simulink model "BuckyWagon_01"  (Simulink 7.5)
settings: Solver=FixedStepDiscrete  StartTime=0.0  StopTime=10.0  RelTol=1e-3
PreLoadFcn:
  | try, eval([bdroot '_setup']); catch, eval('model_setup', ''); end
InitFcn:
  | try, eval([bdroot '_setup']); catch, eval('model_setup', ''); end
undefined symbols (not defined in the file): ECU565, High, Low, miniviewSetup, motohawk_build_version, motohawk_get_faults, motohawk_setup_toolchains, motohawk_trunc_name, motohawk_vardec_config_group, motohawk_vardec_path, tc, True
libraries: MotoHawk_lib x441, simulink x25, motohawk_engine_lib x19, miniview_lib x10, motohawk_control_primitives_lib x8, motohawk_annotations_lib x2
(part 2 of 8)

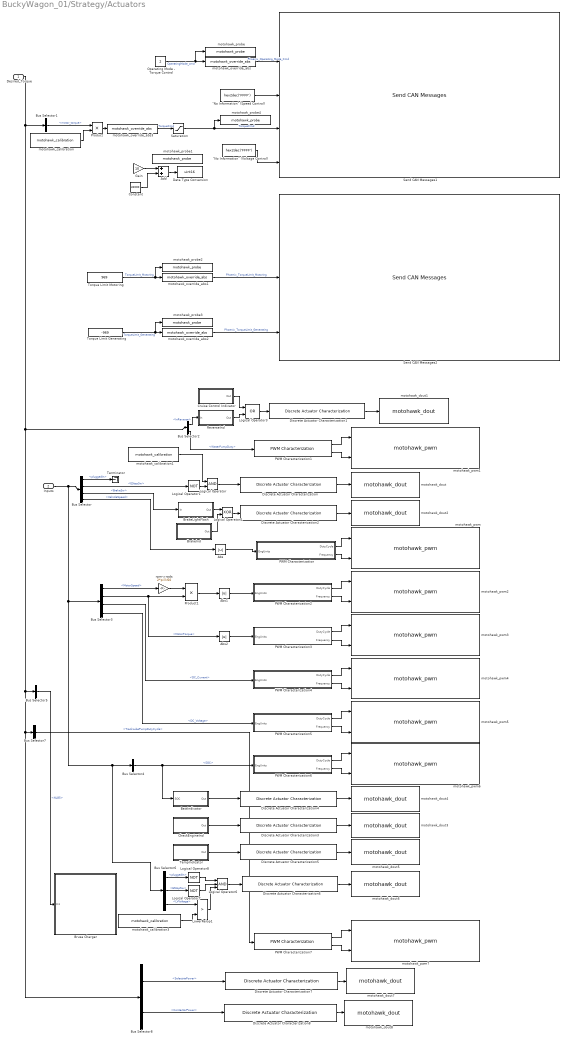
== system BuckyWagon_01/Strategy/Actuators ==
  Desired_Torque : Inport  OutDataType=sfix(16)  OutScaling=2^0
  Inputs : Inport  Port=2  OutDataType=sfix(16)  OutScaling=2^0
  "\"No Information\" (Speed Control)" : Constant  Value=hex2dec('FFFF')  OutDataTypeMode=uint16  OutDataType=sfix(16)  OutScaling=2^0  OutDataTypeStr=uint16
  "\"No Information\" (Voltage Control)" : Constant  Value=hex2dec('FFFF')  OutDataTypeMode=uint16  OutDataType=sfix(16)  OutScaling=2^0  OutDataTypeStr=uint16
  Abs : Abs
  Abs1 : Abs
  Abs2 : Abs
  Add : Sum  OutDataType=fixdt(1, 16)  OutScaling=2^-10
  BattIndicator : Subsystem
  BrakeInd : Subsystem
  BrakeLightFlash : Subsystem
  Brusa Charger : Subsystem  AncestorBlock=motohawk_annotations_lib/Display Image File  mask(Display Image File){image_file='NLG5.jpg'}
      mask prompts: image_file "Image File"
      mask help:
      | Enter an image file on the current MATLAB path to display on this block.
      |
      | Double-clicking this block opens the contents of the subsystem.  Right-click and select 'Mask parameters...' to select a new image file.
      |
      | To use just the mask of this block in a model, but supply your own contents, break the link to the library.
      mask init:
      | try,
      | 	img = imread(image_file);
      | 	motohawk_block_image(gcb, image_file);
      | catch,
      | 	img = imread('image_not_found.jpg');
      | end
      settings: OpenFcn=open_system(gcb,'force');  MoveFcn=motohawk_block_image(gcb, motohawk_get_param_ws(gcb, 'image_file'));
      mask Display: image(img);
  Bus Selector : BusSelector  OutputSignals=Physical.NLG5.pluggedIn,Physical.EStopSw,Physical.BrakeSw,Virtual.VehicleSpeed
  Bus Selector1 : BusSelector  OutputSignals=motor_torque
  Bus Selector2 : BusSelector  OutputSignals=InReverse,WaterPumpDuty
  Bus Selector3 : BusSelector  OutputSignals=Physical.MotorSpeed,Physical.MotorTorque,Physical.DC_Current,Physical.DC_Voltage
  Bus Selector4 : BusSelector  OutputSignals=Virtual.SOC
  Bus Selector5 : BusSelector  OutputSignals=NLG5
  Bus Selector6 : BusSelector  OutputSignals=Physical.NLG5.pluggedIn,Physical.EStopSw,Physical.LVVoltage
  Bus Selector7 : BusSelector  OutputSignals=TrackLubePumpDutyCycle
  Bus Selector8 : BusSelector  OutputSignals=SolectriaPower,ContactorPower
  CheckEngineInd : Subsystem
  Constant : Constant  Value=32000  OutDataType=fixdt(1, 16)  OutScaling=2^0
  Cruise Control Indicator : Subsystem
  Data Type Conversion : DataTypeConversion  OutDataTypeMode=uint16  OutDataType=fixdt(1, 16)  OutScaling=2^0  OutDataTypeStr=uint16
  Discrete Actuator Characterization : motohawk_engine_lib/Discrete Actuator Characterization  SystemSampleTime=-1  prefix='MC_En_'  nam='MC_Enable'  units='bool'  parent_group='Actuators | MC_Enable'  polarity=High-True
  Discrete Actuator Characterization1 : motohawk_engine_lib/Discrete Actuator Characterization  SystemSampleTime=-1  prefix='RevOut_'  nam='ReverseOut'  units='bool'  parent_group='Actuators | Reverse'  polarity=High-True
  Discrete Actuator Characterization2 : motohawk_engine_lib/Discrete Actuator Characterization  SystemSampleTime=-1  prefix='BrkOut_'  nam='Brake_Out'  units='bool'  parent_group='Actuators | Brake'  polarity=High-True
  Discrete Actuator Characterization3 : motohawk_engine_lib/Discrete Actuator Characterization  SystemSampleTime=-1  prefix='ChkEngInd_'  nam='ChkEngInd'  units='bool'  parent_group='Actuators | ChkEngInd'  polarity=High-True
  Discrete Actuator Characterization4 : motohawk_engine_lib/Discrete Actuator Characterization  SystemSampleTime=-1  prefix='BattInd_'  nam='BattInd'  units='bool'  parent_group='Actuators | BattInd'  polarity=High-True
  Discrete Actuator Characterization5 : motohawk_engine_lib/Discrete Actuator Characterization  SystemSampleTime=-1  prefix='TempInd_'  nam='TempInd'  units='bool'  parent_group='Actuators | TempInd'  polarity=High-True
  Discrete Actuator Characterization6 : motohawk_engine_lib/Discrete Actuator Characterization  SystemSampleTime=-1  prefix='ChassisPowerRelayDriver_'  nam='ChassisPowerRelayDriver'  units='bool'  parent_group='Actuators | Chasis Power Relay Driver'  polarity=High-True
  Discrete Actuator Characterization7 : motohawk_engine_lib/Discrete Actuator Characterization  SystemSampleTime=-1  prefix='Solectria_Power_LSD_'  nam='Solectria_Power_LSD'  units='bool'  parent_group='Actuators | Solectria Power LSD'  polarity=Low-True
  Discrete Actuator Characterization8 : motohawk_engine_lib/Discrete Actuator Characterization  SystemSampleTime=-1  prefix='Contactor_Power_LSD_'  nam='Contactor_Power_LSD'  units='bool'  parent_group='Actuators | Contactor Power LSD'  polarity=Low-True
  Gain : Gain  Gain=10  ParameterDataType=fixdt(1, 16)  ParameterScaling=2^0  OutDataType=fixdt(1, 16)  OutScaling=2^0
  Logical Operator : Logic  AllPortsSameDT=off  OutDataTypeMode=boolean  OutDataTypeStr=boolean
  Logical Operator1 : Logic  Operator=NOT  AllPortsSameDT=off  OutDataTypeMode=boolean  OutDataTypeStr=boolean
  Logical Operator3 : Logic  Operator=OR  IconShape=distinctive  AllPortsSameDT=off  OutDataTypeMode=boolean  OutDataTypeStr=boolean
  Logical Operator4 : Logic  Operator=XOR  AllPortsSameDT=off  OutDataTypeMode=boolean  OutDataTypeStr=boolean
  Logical Operator6 : Logic  Inputs=3  AllPortsSameDT=off  OutDataTypeMode=boolean  OutDataTypeStr=boolean
  Logical Operator7 : Logic  Operator=NOT  AllPortsSameDT=off  OutDataTypeMode=boolean  OutDataTypeStr=boolean
  Logical Operator8 : Logic  Operator=NOT  AllPortsSameDT=off  OutDataTypeMode=boolean  OutDataTypeStr=boolean
  LowerRelop1 : RelationalOperator  Operator=>  LogicOutDataTypeMode=boolean  OutDataTypeStr=boolean
  Operating Mode - Torque Control : Constant  Value=2  OutDataType=sfix(16)  OutScaling=2^0
  PWM Characterization : Subsystem  AncestorBlock=motohawk_engine_lib/PWM Characterization  mask(Linear Actuator Characterization){nam='SpeedOut', prefix='SpdOut_', units='mph', parent_group='Actuators | Speed'}
      mask prompts: nam "Name"; parent_group "MotoTune Group"
      mask help:
      | Scales the duty cycle of a PWM signal using a Gain and Offset with a calibratable PWM Frequency.
      | Saturates the converted value around Min and Max values, and converts the signal to the appropriate fixed-point format for use with motoHawk PWM blocks.
      mask init:
      | lbl = ['PWM Characterization: ' nam ];
      | group = [parent_group ' | ' nam];
      settings: RTWSystemCode=Function  RTWFcnNameOpts=Use subsystem name  RTWFileNameOpts=Use function name
      mask Display:
      | patch([0 0 1 1], [0 0.075 0.075 0], [230/255 0/255 0/255])
      | patch([0 0 1 1], [0.025 0.05 0.05 0.025], [150/255 0/255 0/255])
      | patch([0 0 1 1], [0 0.025 0.025 0], [0/255 0/255 0/255])
      | 
      | disp(lbl);
  PWM Characterization1 : motohawk_engine_lib/PWM Characterization  SystemSampleTime=-1  nam='WaterPumpOut'  prefix='WtrPmpOut_'  units='%'  parent_group='Actuators | WaterPump'
  PWM Characterization2 : Subsystem  AncestorBlock=motohawk_engine_lib/PWM Characterization  mask(Linear Actuator Characterization){nam='PowerOut', prefix='PwrOut_', units='W', parent_group='Actuators | Power'}
      mask prompts: nam "Name"; parent_group "MotoTune Group"
      mask help:
      | Scales the duty cycle of a PWM signal using a Gain and Offset with a calibratable PWM Frequency.
      | Saturates the converted value around Min and Max values, and converts the signal to the appropriate fixed-point format for use with motoHawk PWM blocks.
      mask init:
      | lbl = ['PWM Characterization: ' nam ];
      | group = [parent_group ' | ' nam];
      settings: RTWSystemCode=Function  RTWFcnNameOpts=Use subsystem name  RTWFileNameOpts=Use function name
      mask Display:
      | patch([0 0 1 1], [0 0.075 0.075 0], [230/255 0/255 0/255])
      | patch([0 0 1 1], [0.025 0.05 0.05 0.025], [150/255 0/255 0/255])
      | patch([0 0 1 1], [0 0.025 0.025 0], [0/255 0/255 0/255])
      | 
      | disp(lbl);
  PWM Characterization3 : Subsystem  AncestorBlock=motohawk_engine_lib/PWM Characterization  mask(Linear Actuator Characterization){nam='TorqueOut', prefix='TrqOut_', units='Nm', parent_group='Actuators | Torque'}
      mask prompts: nam "Name"; parent_group "MotoTune Group"
      mask help:
      | Scales the duty cycle of a PWM signal using a Gain and Offset with a calibratable PWM Frequency.
      | Saturates the converted value around Min and Max values, and converts the signal to the appropriate fixed-point format for use with motoHawk PWM blocks.
      mask init:
      | lbl = ['PWM Characterization: ' nam ];
      | group = [parent_group ' | ' nam];
      settings: RTWSystemCode=Function  RTWFcnNameOpts=Use subsystem name  RTWFileNameOpts=Use function name
      mask Display:
      | patch([0 0 1 1], [0 0.075 0.075 0], [230/255 0/255 0/255])
      | patch([0 0 1 1], [0.025 0.05 0.05 0.025], [150/255 0/255 0/255])
      | patch([0 0 1 1], [0 0.025 0.025 0], [0/255 0/255 0/255])
      | 
      | disp(lbl);
  PWM Characterization4 : Subsystem  AncestorBlock=motohawk_engine_lib/PWM Characterization  mask(Linear Actuator Characterization){nam='CurrentOut', prefix='CrntOut_', units='A', parent_group='Actuators | Current'}
      mask prompts: nam "Name"; parent_group "MotoTune Group"
      mask help:
      | Scales the duty cycle of a PWM signal using a Gain and Offset with a calibratable PWM Frequency.
      | Saturates the converted value around Min and Max values, and converts the signal to the appropriate fixed-point format for use with motoHawk PWM blocks.
      mask init:
      | lbl = ['PWM Characterization: ' nam ];
      | group = [parent_group ' | ' nam];
      settings: RTWSystemCode=Function  RTWFcnNameOpts=Use subsystem name  RTWFileNameOpts=Use function name
      mask Display:
      | patch([0 0 1 1], [0 0.075 0.075 0], [230/255 0/255 0/255])
      | patch([0 0 1 1], [0.025 0.05 0.05 0.025], [150/255 0/255 0/255])
      | patch([0 0 1 1], [0 0.025 0.025 0], [0/255 0/255 0/255])
      | 
      | disp(lbl);
  PWM Characterization5 : Subsystem  AncestorBlock=motohawk_engine_lib/PWM Characterization  mask(Linear Actuator Characterization){nam='VoltageOut', prefix='VltOut_', units='V', parent_group='Actuators | Voltage'}
      mask prompts: nam "Name"; parent_group "MotoTune Group"
      mask help:
      | Scales the duty cycle of a PWM signal using a Gain and Offset with a calibratable PWM Frequency.
      | Saturates the converted value around Min and Max values, and converts the signal to the appropriate fixed-point format for use with motoHawk PWM blocks.
      mask init:
      | lbl = ['PWM Characterization: ' nam ];
      | group = [parent_group ' | ' nam];
      settings: RTWSystemCode=Function  RTWFcnNameOpts=Use subsystem name  RTWFileNameOpts=Use function name
      mask Display:
      | patch([0 0 1 1], [0 0.075 0.075 0], [230/255 0/255 0/255])
      | patch([0 0 1 1], [0.025 0.05 0.05 0.025], [150/255 0/255 0/255])
      | patch([0 0 1 1], [0 0.025 0.025 0], [0/255 0/255 0/255])
      | 
      | disp(lbl);
  PWM Characterization6 : Subsystem  AncestorBlock=motohawk_engine_lib/PWM Characterization  mask(Linear Actuator Characterization){nam='SOCOut', prefix='SOCOut_', units='%', parent_group='Actuators | SOC'}
      mask prompts: nam "Name"; parent_group "MotoTune Group"
      mask help:
      | Scales the duty cycle of a PWM signal using a Gain and Offset with a calibratable PWM Frequency.
      | Saturates the converted value around Min and Max values, and converts the signal to the appropriate fixed-point format for use with motoHawk PWM blocks.
      mask init:
      | lbl = ['PWM Characterization: ' nam ];
      | group = [parent_group ' | ' nam];
      settings: RTWSystemCode=Function  RTWFcnNameOpts=Use subsystem name  RTWFileNameOpts=Use function name
      mask Display:
      | patch([0 0 1 1], [0 0.075 0.075 0], [230/255 0/255 0/255])
      | patch([0 0 1 1], [0.025 0.05 0.05 0.025], [150/255 0/255 0/255])
      | patch([0 0 1 1], [0 0.025 0.025 0], [0/255 0/255 0/255])
      | 
      | disp(lbl);
  PWM Characterization7 : motohawk_engine_lib/PWM Characterization  SystemSampleTime=-1  nam='TrackLubePumpOut'  prefix='TrackLubePumpOut_'  units='%'  parent_group='Actuators | TrackLubePump'
  Product : Product  OutDataType=sfix(16)  OutScaling=2^0  RndMeth=Zero
  Product1 : Product  OutDataType=sfix(16)  OutScaling=2^0  RndMeth=Zero
  ReverseInd : Subsystem
  Saturation : Saturate  UpperLimit=+3200  LowerLimit=-3200  OutDataType=fixdt(1, 16)  OutScaling=2^0
  Send CAN Messages1 : MotoHawk_lib/CAN Blocks/Send CAN Messages  bus=-2  nam='CAN_1'  msgl=J1939_F9_Control1  pace=5  labelwires=off
  Send CAN Messages2 : MotoHawk_lib/CAN Blocks/Send CAN Messages  bus=-2  nam='CAN_1'  msgl=J1939_F9_Control2  pace=5  labelwires=off
  TempIndicator : Subsystem
  Terminator : Terminator
  Torque Limit Generating : Constant  Value=-969  OutDataType=sfix(16)  OutScaling=2^0
  Torque Limit Motoring : Constant  Value=969  OutDataType=sfix(16)  OutScaling=2^0
  motohawk_calibration : MotoHawk_lib/Calibration & Probing Blocks/motohawk_calibration  nam='MaxTorque'  val=120  storage=Calibration  show_more=on  name_source=Use Parameter  data_type=Inherit from 'Default Value'  read_level=1  write_level=1  ovr_cals=on  view_as=Number  enum_struct={'Disabled', 'Enabled'}  vector_style=Wide Row  use_help_units=off  help=''  units=''  use_header_enum=off  row_header_enum={}  col_header_enum={}  use_min_max=off  min_val=-inf  max_val=inf  use_precision=off  precision=''  gain=1  offset=0  exp=1  use_mototune_group=on  mototune_group='Actuators | Phoenix'
  motohawk_calibration1 : MotoHawk_lib/Calibration & Probing Blocks/motohawk_calibration  nam='MC_Enable'  val=0  storage=Calibration  show_more=on  name_source=Use Parameter  data_type=int8  read_level=1  write_level=1  ovr_cals=on  view_as=Enumeration  enum_struct={'Disabled', 'Enabled'}  vector_style=Wide Row  use_help_units=off  help=''  units=''  use_header_enum=off  row_header_enum={}  col_header_enum={}  use_min_max=off  min_val=-inf  max_val=inf  use_precision=off  precision=''  gain=1  offset=0  exp=1  use_mototune_group=off  mototune_group=motohawk_vardec_path(gcb)
  motohawk_calibration3 : MotoHawk_lib/Calibration & Probing Blocks/motohawk_calibration  nam='ChassisPower_MinSysVolt'  val=12  storage=Calibration  show_more=on  name_source=Use Parameter  data_type=Inherit from 'Default Value'  read_level=1  write_level=1  ovr_cals=on  view_as=Number  enum_struct={'Disabled', 'Enabled'}  vector_style=Wide Row  use_help_units=on  help='Minimum system voltage to turn on chassis power'  units='V'  use_header_enum=off  row_header_enum={}  col_header_enum={}  use_min_max=on  min_val=2  max_val=20  use_precision=on  precision='1.0'  gain=1  offset=0  exp=1  use_mototune_group=on  mototune_group='ESled_11 | Actuators | Chassis Power Relay Driver'
  motohawk_dout : MotoHawk_lib/Digital I//O Blocks/motohawk_dout  resource_name=[]  text_resource=(None)  target=ECU565-128  use_diag=off  use_vardec=on  nam='MC_Enable_Pin'  read_level=1  write_level=1  group='System | I/O Pins | Outputs Config'
  motohawk_dout1 : MotoHawk_lib/Digital I//O Blocks/motohawk_dout  resource_name=[]  text_resource=(None)  target=ECU565-128  use_diag=off  use_vardec=on  nam='ReverseOut_Pin'  read_level=1  write_level=1  group='System | I/O Pins | Outputs Config'
  motohawk_dout2 : MotoHawk_lib/Digital I//O Blocks/motohawk_dout  resource_name=[]  text_resource=(None)  target=ECU565-128  use_diag=off  use_vardec=on  nam='BrakeOut_Pin'  read_level=1  write_level=1  group='System | I/O Pins | Outputs Config'
  motohawk_dout3 : MotoHawk_lib/Digital I//O Blocks/motohawk_dout  resource_name=[]  text_resource=(None)  target=ECU565-128  use_diag=off  use_vardec=on  nam='ChkEngInd_Pin'  read_level=1  write_level=1  group='System | I/O Pins | Outputs Config'
  motohawk_dout4 : MotoHawk_lib/Digital I//O Blocks/motohawk_dout  resource_name=[]  text_resource=(None)  target=ECU565-128  use_diag=off  use_vardec=on  nam='BattInd_Pin'  read_level=1  write_level=1  group='System | I/O Pins | Outputs Config'
  motohawk_dout5 : MotoHawk_lib/Digital I//O Blocks/motohawk_dout  resource_name=[]  text_resource=(None)  target=ECU565-128  use_diag=off  use_vardec=on  nam='TempInd_Pin'  read_level=1  write_level=1  group='System | I/O Pins | Outputs Config'
  motohawk_dout6 : MotoHawk_lib/Digital I//O Blocks/motohawk_dout  resource_name=[]  text_resource=(None)  target=ECU565-128  use_diag=off  use_vardec=on  nam='ChassisPowerRelayDriver_Pin'  read_level=1  write_level=1  group='System | I/O Pins | Outputs Config'
  motohawk_dout7 : MotoHawk_lib/Digital I//O Blocks/motohawk_dout  resource_name=[]  text_resource=(None)  target=ECU565-128  use_diag=off  use_vardec=on  nam='SolectriaPowerLSD_Pin'  read_level=1  write_level=1  group='System | I/O Pins | Outputs Config'
  motohawk_dout8 : MotoHawk_lib/Digital I//O Blocks/motohawk_dout  resource_name=[]  text_resource=(None)  target=ECU565-128  use_diag=off  use_vardec=on  nam='ContactorPowerLSD_Pin'  read_level=1  write_level=1  group='System | I/O Pins | Outputs Config'
  motohawk_override_abs : MotoHawk_lib/Calibration & Probing Blocks/motohawk_override_abs  SystemSampleTime=-1  parent_name='Override_Absolute'  parent_val=0  show_more=on  name_source=Use Output Wire Name  parent_read_level=1  parent_override_level=1  view_as=Number  enum_struct={'Disabled', 'Enabled'}  use_help_units=off  parent_help=''  parent_units=''  use_min_max=off  parent_min=-inf  parent_max=inf  use_precision=off  parent_precision=''  parent_gain=1  parent_offset=0  parent_exp=1  use_mototune_group=on  parent_group='Actuators | Phoenix'
  motohawk_override_abs1 : MotoHawk_lib/Calibration & Probing Blocks/motohawk_override_abs  SystemSampleTime=-1  parent_name='Override_Absolute'  parent_val=0  show_more=on  name_source=Use Output Wire Name  parent_read_level=1  parent_override_level=1  view_as=Number  enum_struct={'Disabled', 'Enabled'}  use_help_units=off  parent_help=''  parent_units=''  use_min_max=off  parent_min=-inf  parent_max=inf  use_precision=off  parent_precision=''  parent_gain=1  parent_offset=0  parent_exp=1  use_mototune_group=on  parent_group='Actuators | Phoenix'
  motohawk_override_abs2 : MotoHawk_lib/Calibration & Probing Blocks/motohawk_override_abs  SystemSampleTime=-1  parent_name='Override_Absolute'  parent_val=0  show_more=on  name_source=Use Output Wire Name  parent_read_level=1  parent_override_level=1  view_as=Number  enum_struct={'Disabled', 'Enabled'}  use_help_units=off  parent_help=''  parent_units=''  use_min_max=off  parent_min=-inf  parent_max=inf  use_precision=off  parent_precision=''  parent_gain=1  parent_offset=0  parent_exp=1  use_mototune_group=on  parent_group='Actuators | Phoenix'
  motohawk_override_abs3 : MotoHawk_lib/Calibration & Probing Blocks/motohawk_override_abs  SystemSampleTime=-1  parent_name='TorqueControl'  parent_val=0  show_more=on  name_source=Use Parameter  parent_read_level=1  parent_override_level=1  view_as=Number  enum_struct={'Disabled', 'Enabled'}  use_help_units=off  parent_help=''  parent_units=''  use_min_max=off  parent_min=-inf  parent_max=inf  use_precision=off  parent_precision=''  parent_gain=1  parent_offset=0  parent_exp=1  use_mototune_group=on  parent_group='Actuators | Phoenix'
  motohawk_probe : MotoHawk_lib/Calibration & Probing Blocks/motohawk_probe  nam='Phoenix_Operating_Mode_Command'  show_more=on  name_source=Use Parameter  read_level=1  view_as=Number  enum_struct={'Disabled', 'Enabled'}  vector_style=Wide Row  use_help_units=off  help=''  units=''  use_header_enum=off  row_header_enum={}  col_header_enum={}  use_precision=off  precision=''  gain=1  offset=0  exp=1  use_mototune_group=on  mototune_group='Actuators | Phoenix'
  motohawk_probe1 : MotoHawk_lib/Calibration & Probing Blocks/motohawk_probe  nam='Phoenix_TorqueCmd_integer'  show_more=on  name_source=Use Parameter  read_level=1  view_as=Number  enum_struct={'Disabled', 'Enabled'}  vector_style=Wide Row  use_help_units=off  help=''  units=''  use_header_enum=off  row_header_enum={}  col_header_enum={}  use_precision=off  precision=''  gain=1  offset=0  exp=1  use_mototune_group=on  mototune_group='Actuators | Phoenix'
  motohawk_probe2 : MotoHawk_lib/Calibration & Probing Blocks/motohawk_probe  nam='Phoenix_TorqueLimit_Motoring'  show_more=on  name_source=Use Parameter  read_level=1  view_as=Number  enum_struct={'Disabled', 'Enabled'}  vector_style=Wide Row  use_help_units=off  help=''  units=''  use_header_enum=off  row_header_enum={}  col_header_enum={}  use_precision=off  precision=''  gain=1  offset=0  exp=1  use_mototune_group=on  mototune_group='Actuators | Phoenix'
  motohawk_probe3 : MotoHawk_lib/Calibration & Probing Blocks/motohawk_probe  nam='Phoenix_TorqueLimit_Generating'  show_more=on  name_source=Use Parameter  read_level=1  view_as=Number  enum_struct={'Disabled', 'Enabled'}  vector_style=Wide Row  use_help_units=off  help=''  units=''  use_header_enum=off  row_header_enum={}  col_header_enum={}  use_precision=off  precision=''  gain=1  offset=0  exp=1  use_mototune_group=on  mototune_group='Actuators | Phoenix'
  motohawk_probe4 : MotoHawk_lib/Calibration & Probing Blocks/motohawk_probe  nam='Phoenix_TorqueCmd_final'  show_more=on  name_source=Use Parameter  read_level=1  view_as=Number  enum_struct={'Disabled', 'Enabled'}  vector_style=Wide Row  use_help_units=off  help=''  units=''  use_header_enum=off  row_header_enum={}  col_header_enum={}  use_precision=off  precision=''  gain=1  offset=0  exp=1  use_mototune_group=on  mototune_group='Actuators | Phoenix'
  motohawk_pwm : MotoHawk_lib/Analog I//O Blocks/motohawk_pwm  res_name=[]  text_resource=(None)  code_resource=NONE  val_resource=-1  target=ECU565-128  resource_enum_str=(None)=-1,H1=1,H2=10,FINJ1=12,FINJ2=13,FINJ3=14,FINJ4=15,FINJ5=16,FINJ6=17,FINJ7=18,FINJ8=19,FINJ9=20,FINJ10=21,FINJ11=22,FINJ12=23,TACH=24,LSD1=25,LSD2=26,LSD3=27,LSD4=28,LSD5=29,LSD6=30,LSD7=31,LSD8=32,LSD9=33,LSD10=34,EST 1=36,EST 2=37,EST 3=38,EST 4=39,EST 5=40,EST 6=41,EST 7=42,EST 8=43,EST 9=44,EST 10=45,EST 11=46,EST 12=47,EST 13=48,EST 14=49,EST 15=50,EST 16=51,H3=107  freq_mode=-1  min_freq=2  use_max_freq=off  max_freq=42949672.96  use_enable=off  use_brake=off  output_current=off  output_fault_status=off  use_child=off  use_vardec=on  nam='SpeedOut_Pin'  read_level=1  write_level=1  group='System | I/O Pins | Outputs Config'
  motohawk_pwm1 : MotoHawk_lib/Analog I//O Blocks/motohawk_pwm  res_name=[]  text_resource=(None)  code_resource=NONE  val_resource=-1  target=ECU565-128  resource_enum_str=(None)=-1,H1=1,H2=10,FINJ1=12,FINJ2=13,FINJ3=14,FINJ4=15,FINJ5=16,FINJ6=17,FINJ7=18,FINJ8=19,FINJ9=20,FINJ10=21,FINJ11=22,FINJ12=23,TACH=24,LSD1=25,LSD2=26,LSD3=27,LSD4=28,LSD5=29,LSD6=30,LSD7=31,LSD8=32,LSD9=33,LSD10=34,EST 1=36,EST 2=37,EST 3=38,EST 4=39,EST 5=40,EST 6=41,EST 7=42,EST 8=43,EST 9=44,EST 10=45,EST 11=46,EST 12=47,EST 13=48,EST 14=49,EST 15=50,EST 16=51,H3=107  freq_mode=-1  min_freq=2  use_max_freq=off  max_freq=42949672.96  use_enable=off  use_brake=off  output_current=off  output_fault_status=off  use_child=off  use_vardec=on  nam='WaterPump_Pin'  read_level=1  write_level=1  group='System | I/O Pins | Outputs Config'
  motohawk_pwm2 : MotoHawk_lib/Analog I//O Blocks/motohawk_pwm  res_name=[]  text_resource=(None)  code_resource=NONE  val_resource=-1  target=ECU565-128  resource_enum_str=(None)=-1,H1=1,H2=10,FINJ1=12,FINJ2=13,FINJ3=14,FINJ4=15,FINJ5=16,FINJ6=17,FINJ7=18,FINJ8=19,FINJ9=20,FINJ10=21,FINJ11=22,FINJ12=23,TACH=24,LSD1=25,LSD2=26,LSD3=27,LSD4=28,LSD5=29,LSD6=30,LSD7=31,LSD8=32,LSD9=33,LSD10=34,EST 1=36,EST 2=37,EST 3=38,EST 4=39,EST 5=40,EST 6=41,EST 7=42,EST 8=43,EST 9=44,EST 10=45,EST 11=46,EST 12=47,EST 13=48,EST 14=49,EST 15=50,EST 16=51,H3=107  freq_mode=-1  min_freq=2  use_max_freq=off  max_freq=42949672.96  use_enable=off  use_brake=off  output_current=off  output_fault_status=off  use_child=off  use_vardec=on  nam='PowerOut_Pin'  read_level=1  write_level=1  group='System | I/O Pins | Outputs Config'
  motohawk_pwm3 : MotoHawk_lib/Analog I//O Blocks/motohawk_pwm  res_name=[]  text_resource=(None)  code_resource=NONE  val_resource=-1  target=ECU565-128  resource_enum_str=(None)=-1,H1=1,H2=10,FINJ1=12,FINJ2=13,FINJ3=14,FINJ4=15,FINJ5=16,FINJ6=17,FINJ7=18,FINJ8=19,FINJ9=20,FINJ10=21,FINJ11=22,FINJ12=23,TACH=24,LSD1=25,LSD2=26,LSD3=27,LSD4=28,LSD5=29,LSD6=30,LSD7=31,LSD8=32,LSD9=33,LSD10=34,EST 1=36,EST 2=37,EST 3=38,EST 4=39,EST 5=40,EST 6=41,EST 7=42,EST 8=43,EST 9=44,EST 10=45,EST 11=46,EST 12=47,EST 13=48,EST 14=49,EST 15=50,EST 16=51,H3=107  freq_mode=-1  min_freq=2  use_max_freq=off  max_freq=42949672.96  use_enable=off  use_brake=off  output_current=off  output_fault_status=off  use_child=off  use_vardec=on  nam='TorqueOut_Pin'  read_level=1  write_level=1  group='System | I/O Pins | Outputs Config'
  motohawk_pwm4 : MotoHawk_lib/Analog I//O Blocks/motohawk_pwm  res_name=[]  text_resource=(None)  code_resource=NONE  val_resource=-1  target=ECU565-128  resource_enum_str=(None)=-1,H1=1,H2=10,FINJ1=12,FINJ2=13,FINJ3=14,FINJ4=15,FINJ5=16,FINJ6=17,FINJ7=18,FINJ8=19,FINJ9=20,FINJ10=21,FINJ11=22,FINJ12=23,TACH=24,LSD1=25,LSD2=26,LSD3=27,LSD4=28,LSD5=29,LSD6=30,LSD7=31,LSD8=32,LSD9=33,LSD10=34,EST 1=36,EST 2=37,EST 3=38,EST 4=39,EST 5=40,EST 6=41,EST 7=42,EST 8=43,EST 9=44,EST 10=45,EST 11=46,EST 12=47,EST 13=48,EST 14=49,EST 15=50,EST 16=51,H3=107  freq_mode=-1  min_freq=2  use_max_freq=off  max_freq=42949672.96  use_enable=off  use_brake=off  output_current=off  output_fault_status=off  use_child=off  use_vardec=on  nam='CurrentOut_Pin'  read_level=1  write_level=1  group='System | I/O Pins | Outputs Config'
  motohawk_pwm5 : MotoHawk_lib/Analog I//O Blocks/motohawk_pwm  res_name=[]  text_resource=(None)  code_resource=NONE  val_resource=-1  target=ECU565-128  resource_enum_str=(None)=-1,H1=1,H2=10,FINJ1=12,FINJ2=13,FINJ3=14,FINJ4=15,FINJ5=16,FINJ6=17,FINJ7=18,FINJ8=19,FINJ9=20,FINJ10=21,FINJ11=22,FINJ12=23,TACH=24,LSD1=25,LSD2=26,LSD3=27,LSD4=28,LSD5=29,LSD6=30,LSD7=31,LSD8=32,LSD9=33,LSD10=34,EST 1=36,EST 2=37,EST 3=38,EST 4=39,EST 5=40,EST 6=41,EST 7=42,EST 8=43,EST 9=44,EST 10=45,EST 11=46,EST 12=47,EST 13=48,EST 14=49,EST 15=50,EST 16=51,H3=107  freq_mode=-1  min_freq=2  use_max_freq=off  max_freq=42949672.96  use_enable=off  use_brake=off  output_current=off  output_fault_status=off  use_child=off  use_vardec=on  nam='VoltageOut_Pin'  read_level=1  write_level=1  group='System | I/O Pins | Outputs Config'
  motohawk_pwm6 : MotoHawk_lib/Analog I//O Blocks/motohawk_pwm  res_name=[]  text_resource=(None)  code_resource=NONE  val_resource=-1  target=ECU565-128  resource_enum_str=(None)=-1,H1=1,H2=10,FINJ1=12,FINJ2=13,FINJ3=14,FINJ4=15,FINJ5=16,FINJ6=17,FINJ7=18,FINJ8=19,FINJ9=20,FINJ10=21,FINJ11=22,FINJ12=23,TACH=24,LSD1=25,LSD2=26,LSD3=27,LSD4=28,LSD5=29,LSD6=30,LSD7=31,LSD8=32,LSD9=33,LSD10=34,EST 1=36,EST 2=37,EST 3=38,EST 4=39,EST 5=40,EST 6=41,EST 7=42,EST 8=43,EST 9=44,EST 10=45,EST 11=46,EST 12=47,EST 13=48,EST 14=49,EST 15=50,EST 16=51,H3=107  freq_mode=-1  min_freq=2  use_max_freq=off  max_freq=42949672.96  use_enable=off  use_brake=off  output_current=off  output_fault_status=off  use_child=off  use_vardec=on  nam='SOCOut_Pin'  read_level=1  write_level=1  group='System | I/O Pins | Outputs Config'
  motohawk_pwm7 : MotoHawk_lib/Analog I//O Blocks/motohawk_pwm  res_name=[]  text_resource=(None)  code_resource=NONE  val_resource=-1  target=ECU565-128  resource_enum_str=(None)=-1,H1=1,H2=10,FINJ1=12,FINJ2=13,FINJ3=14,FINJ4=15,FINJ5=16,FINJ6=17,FINJ7=18,FINJ8=19,FINJ9=20,FINJ10=21,FINJ11=22,FINJ12=23,TACH=24,LSD1=25,LSD2=26,LSD3=27,LSD4=28,LSD5=29,LSD6=30,LSD7=31,LSD8=32,LSD9=33,LSD10=34,EST 1=36,EST 2=37,EST 3=38,EST 4=39,EST 5=40,EST 6=41,EST 7=42,EST 8=43,EST 9=44,EST 10=45,EST 11=46,EST 12=47,EST 13=48,EST 14=49,EST 15=50,EST 16=51,H3=107  freq_mode=-1  min_freq=2  use_max_freq=off  max_freq=42949672.96  use_enable=off  use_brake=off  output_current=off  output_fault_status=off  use_child=off  use_vardec=on  nam='TrackLubePump_Pin'  read_level=1  write_level=1  group='System | I/O Pins | Outputs Config'
  rpm->rads : Gain  Gain=2*pi()/60  ParameterDataType=sfix(16)  ParameterScaling=2^0  OutDataType=sfix(16)  OutScaling=2^0
  wires:
  motohawk_override_abs/1 -> Send CAN Messages1/2  "Phoenix_Operating_Mode_Cmd"
  Operating Mode - Torque Control/1 -> motohawk_override_abs/1, motohawk_probe/1  "OperatingMode_cmd"
  motohawk_calibration/1 -> Product/2
  Product/1 -> motohawk_override_abs3/1
  Discrete Actuator Characterization/1 -> motohawk_dout/1
  Inputs/1 -> Bus Selector/1, Bus Selector3/1, Bus Selector4/1, Bus Selector6/1
  Logical Operator/1 -> Discrete Actuator Characterization/1
  motohawk_calibration1/1 -> Logical Operator/1
  Bus Selector/2 -> Logical Operator1/1  "<EStopSw>"
  Discrete Actuator Characterization1/1 -> motohawk_dout1/1
  Discrete Actuator Characterization2/1 -> motohawk_dout2/1
  PWM Characterization/1(DutyCycle) -> motohawk_pwm/1
  PWM Characterization/2(Frequency) -> motohawk_pwm/2
  Bus Selector/3 -> BrakeLightFlash/1(In)  "<BrakeSw>"
  Desired_Torque/1 -> Bus Selector1/1, Bus Selector2/1, Bus Selector5/1, Bus Selector7/1, Bus Selector8/1
  Bus Selector1/1 -> Product/1  "<motor_torque>"
  Bus Selector/4 -> Abs/1  "<VehicleSpeed>"
  PWM Characterization1/1 -> motohawk_pwm1/1
  PWM Characterization1/2 -> motohawk_pwm1/2
  Bus Selector2/2 -> PWM Characterization1/1  "<WaterPumpDuty>"
  Logical Operator1/1 -> Logical Operator/2
  PWM Characterization2/1(DutyCycle) -> motohawk_pwm2/1
  PWM Characterization2/2(Frequency) -> motohawk_pwm2/2
  PWM Characterization3/1(DutyCycle) -> motohawk_pwm3/1
  PWM Characterization3/2(Frequency) -> motohawk_pwm3/2
  Bus Selector3/1 -> rpm->rads/1  "<MotorSpeed>"
  rpm->rads/1 -> Product1/1
  Bus Selector3/2 -> Product1/2, Abs2/1  "<MotorTorque>"
  Product1/1 -> Abs1/1
  Discrete Actuator Characterization3/1 -> motohawk_dout3/1
  CheckEngineInd/1(Out) -> Discrete Actuator Characterization3/1
  Discrete Actuator Characterization4/1 -> motohawk_dout4/1
  PWM Characterization4/1(DutyCycle) -> motohawk_pwm4/1
  PWM Characterization4/2(Frequency) -> motohawk_pwm4/2
  PWM Characterization5/1(DutyCycle) -> motohawk_pwm5/1
  PWM Characterization5/2(Frequency) -> motohawk_pwm5/2
  Discrete Actuator Characterization5/1 -> motohawk_dout5/1
  TempIndicator/1(Out) -> Discrete Actuator Characterization5/1
  Bus Selector3/3 -> PWM Characterization4/1(EngUnits)  "<DC_Current>"
  Bus Selector3/4 -> PWM Characterization5/1(EngUnits)  "<DC_Voltage>"
  BattIndicator/1(Out) -> Discrete Actuator Characterization4/1
  Bus Selector4/1 -> BattIndicator/1(SOC), PWM Characterization6/1(EngUnits)  "<SOC>"
  PWM Characterization6/1(DutyCycle) -> motohawk_pwm6/1
  PWM Characterization6/2(Frequency) -> motohawk_pwm6/2
  Abs/1 -> PWM Characterization/1(EngUnits)
  Abs1/1 -> PWM Characterization2/1(EngUnits)
  Abs2/1 -> PWM Characterization3/1(EngUnits)
  Bus Selector2/1 -> ReverseInd/1(In)  "<InReverse>"
  Cruise Control Indicator/1(Out) -> Logical Operator3/1
  ReverseInd/1(Out) -> Logical Operator3/2
  Logical Operator3/1 -> Discrete Actuator Characterization1/1
  Bus Selector5/1 -> Brusa Charger/1(In1)  "<NLG5>"
  BrakeLightFlash/1(Out) -> Logical Operator4/1
  BrakeInd/1(Out) -> Logical Operator4/2
  Logical Operator4/1 -> Discrete Actuator Characterization2/1
  Bus Selector6/1 -> Logical Operator8/1  "<pluggedIn>"
  Bus Selector6/2 -> Logical Operator7/1  "<EStopSw>"
  Logical Operator6/1 -> Discrete Actuator Characterization6/1
  Logical Operator8/1 -> Logical Operator6/1
  Logical Operator7/1 -> Logical Operator6/2
  motohawk_calibration3/1 -> LowerRelop1/2
  Bus Selector6/3 -> LowerRelop1/1  "<LVVoltage>"
  LowerRelop1/1 -> Logical Operator6/3
  Discrete Actuator Characterization6/1 -> motohawk_dout6/1
  PWM Characterization7/1 -> motohawk_pwm7/1
  PWM Characterization7/2 -> motohawk_pwm7/2
  Bus Selector7/1 -> PWM Characterization7/1  "<TrackLubePumpDutyCycle>"
  Discrete Actuator Characterization8/1 -> motohawk_dout8/1
  Discrete Actuator Characterization7/1 -> motohawk_dout7/1
  Bus Selector8/1 -> Discrete Actuator Characterization7/1  "<SolectriaPower>"
  Bus Selector8/2 -> Discrete Actuator Characterization8/1  "<ContactorPower>"
  Bus Selector/1 -> Terminator/1  "<pluggedIn>"
  "\"No Information\" (Speed Control)"/1 -> Send CAN Messages1/3
  "\"No Information\" (Voltage Control)"/1 -> Send CAN Messages1/5
  motohawk_override_abs3/1 -> Saturation/1  "TorqueCmd"
  Saturation/1 -> Send CAN Messages1/4, motohawk_probe4/1  "TorqueCmd"
  motohawk_override_abs1/1 -> Send CAN Messages2/2  "Phoenix_TorqueLimit_Motoring"
  Torque Limit Motoring/1 -> motohawk_probe2/1, motohawk_override_abs1/1  "TorqueLimit_Motoring"
  motohawk_override_abs2/1 -> Send CAN Messages2/3  "Phoenix_TorqueLimit_Generating"
  Torque Limit Generating/1 -> motohawk_override_abs2/1, motohawk_probe3/1  "TorqueLimit_Generating"
  Gain/1 -> Add/1
  Constant/1 -> Add/2
  Add/1 -> Data Type Conversion/1

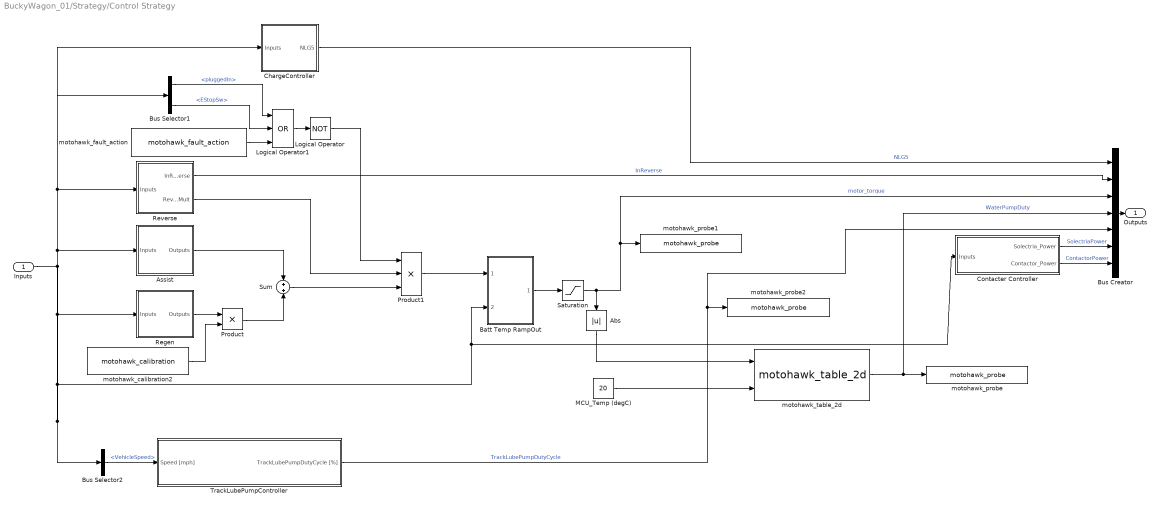
== system BuckyWagon_01/Strategy/Control Strategy ==
  Inputs : Inport  OutDataType=sfix(16)  OutScaling=2^0
  Abs : Abs
  Assist : Subsystem  TreatAsAtomicUnit=on
  Batt Temp RampOut : Subsystem
  Bus Creator : BusCreator  Inputs=7
  Bus Selector1 : BusSelector  OutputSignals=Physical.NLG5.pluggedIn,Physical.EStopSw
  Bus Selector2 : BusSelector  OutputSignals=Virtual.VehicleSpeed
  ChargeController : Subsystem  TreatAsAtomicUnit=on
  Contacter Controller : Subsystem
  Logical Operator : Logic  Operator=NOT  AllPortsSameDT=off  OutDataTypeMode=boolean  OutDataTypeStr=boolean
  Logical Operator1 : Logic  Operator=OR  Inputs=3  AllPortsSameDT=off  OutDataTypeMode=boolean  OutDataTypeStr=boolean
  MCU_Temp (degC) : Constant  Value=20  OutDataType=fixdt(1, 16)  OutScaling=2^0
  Product : Product  OutDataType=sfix(16)  OutScaling=2^0  RndMeth=Zero
  Product1 : Product  Inputs=3  OutDataType=sfix(16)  OutScaling=2^0  RndMeth=Zero
  Regen : Subsystem  TreatAsAtomicUnit=on
  Reverse : Subsystem  TreatAsAtomicUnit=on
  Saturation : Saturate  UpperLimit=1  LowerLimit=-1
  Sum : Sum  OutDataType=sfix(16)  OutScaling=2^0
  TrackLubePumpController : Subsystem  TreatAsAtomicUnit=on
  motohawk_calibration2 : MotoHawk_lib/Calibration & Probing Blocks/motohawk_calibration  nam='Regen_Enable'  val=0  storage=Calibration  show_more=on  name_source=Use Parameter  data_type=Inherit from 'Default Value'  read_level=1  write_level=1  ovr_cals=on  view_as=Number  enum_struct={'Disabled', 'Enabled'}  vector_style=Wide Row  use_help_units=on  help='Enables Regen Braking'  units=''  use_header_enum=off  row_header_enum={}  col_header_enum={}  use_min_max=off  min_val=0  max_val=1  use_precision=on  precision='1.0'  gain=1  offset=0  exp=1  use_mototune_group=off  mototune_group=motohawk_vardec_path(gcb)
  motohawk_fault_action : MotoHawk_lib/Fault Management Blocks/motohawk_fault_action  nam='DisableDrive'  output_status=on  eval_nam=DisableDrive
  motohawk_probe : MotoHawk_lib/Calibration & Probing Blocks/motohawk_probe  nam='WaterPumpDuty'  show_more=off  name_source=Use Parameter  read_level=1  view_as=Number  enum_struct={'Disabled', 'Enabled'}  vector_style=Wide Row  use_help_units=off  help=''  units=''  use_header_enum=off  row_header_enum={}  col_header_enum={}  use_precision=off  precision=''  gain=1  offset=0  exp=1  use_mototune_group=off  mototune_group=motohawk_vardec_path(gcb)
  motohawk_probe1 : MotoHawk_lib/Calibration & Probing Blocks/motohawk_probe  nam='motor_Torque'  show_more=on  name_source=Use Parameter  read_level=1  view_as=Number  enum_struct={'Disabled', 'Enabled'}  vector_style=Wide Row  use_help_units=off  help=''  units=''  use_header_enum=off  row_header_enum={}  col_header_enum={}  use_precision=on  precision='1.3'  gain=1  offset=0  exp=1  use_mototune_group=off  mototune_group=motohawk_vardec_path(gcb)
  motohawk_probe2 : MotoHawk_lib/Calibration & Probing Blocks/motohawk_probe  nam='TrackLubePumpDutyCycle'  show_more=on  name_source=Use Parameter  read_level=1  view_as=Number  enum_struct={'Disabled', 'Enabled'}  vector_style=Wide Row  use_help_units=off  help=''  units=''  use_header_enum=off  row_header_enum={}  col_header_enum={}  use_precision=on  precision='1.3'  gain=1  offset=0  exp=1  use_mototune_group=off  mototune_group=motohawk_vardec_path(gcb)
  motohawk_table_2d : MotoHawk_lib/Lookup Tables/motohawk_table_2d  SystemSampleTime=-1  nam='WaterPumpDutyMap'  row_nam='MotorTorque'  col_nam='MCUTemp'  row_breakpoint_data=0:0.1:1  col_breakpoint_data=0:10:100  table_data=ones(11,11)  show_more=off  row_bp_data_type=Inherit from 'Row Breakpoint Data'  col_bp_data_type=Inherit from 'Column Breakpoint Data'  bp_storage=Constant  table_data_type=Inherit from 'Table Data'  storage=NonAdaptive  read_level=1  write_level=1  ovr_cals=on  use_help=off  help=''  row_bp_units=''  col_bp_units=''  table_units=''  use_min_max=off  row_bp_min_val=-inf  row_bp_max_val=inf  col_bp_min_val=-inf  col_bp_max_val=inf  min_val=-inf  max_val=inf  use_precision=off  use_row_breakpoint=off  rb_precision=''  rb_gain=1  rb_offset=0  rb_exp=1  use_col_breakpoint=off  cb_precision=''  cb_gain=1  cb_offset=0  cb_exp=1  use_table=off  t_precision=''  t_gain=1  t_offset=0  t_exp=1  use_links=off  row_input_name=''  col_input_name=''  output_name=''  use_mototune_group=off  mototune_group=motohawk_vardec_path(gcb)
  Outputs : Outport  OutDataType=sfix(16)  OutScaling=2^0
  wires:
  Inputs/1 -> Assist/1(Inputs), Reverse/1(Inputs), Bus Selector1/1, Regen/1(Inputs), ChargeController/1(Inputs), Bus Selector2/1, Batt Temp RampOut/2(Sensors), Contacter Controller/1(Inputs)
  Saturation/1 -> motohawk_probe1/1, Bus Creator/3, Abs/1  "motor_torque"
  Regen/1(Outputs) -> Product/1
  motohawk_calibration2/1 -> Product/2
  Assist/1(Outputs) -> Sum/1
  Batt Temp RampOut/1(Torque_Out) -> Saturation/1
  Product/1 -> Sum/2
  Reverse/2(ReverseMult) -> Product1/2
  Product1/1 -> Batt Temp RampOut/1(Torque_In)
  Sum/1 -> Product1/3
  Logical Operator/1 -> Product1/1
  Reverse/1(InReverse) -> Bus Creator/2  "InReverse"
  Bus Creator/1 -> Outputs/1
  Abs/1 -> motohawk_table_2d/1
  MCU_Temp (degC)/1 -> motohawk_table_2d/2
  motohawk_table_2d/1 -> motohawk_probe/1, Bus Creator/4  "WaterPumpDuty"
  Bus Selector1/2 -> Logical Operator1/2  "<EStopSw>"
  motohawk_fault_action/1 -> Logical Operator1/3
  Logical Operator1/1 -> Logical Operator/1
  Bus Selector1/1 -> Logical Operator1/1  "<pluggedIn>"
  ChargeController/1(NLG5) -> Bus Creator/1  "NLG5"
  Bus Selector2/1 -> TrackLubePumpController/1(Speed [mph])  "<VehicleSpeed>"
  TrackLubePumpController/1(TrackLubePumpDutyCycle [%]) -> Bus Creator/5, motohawk_probe2/1  "TrackLubePumpDutyCycle"
  Contacter Controller/1(Solectria_Power) -> Bus Creator/6  "SolectriaPower"
  Contacter Controller/2(Contactor_Power) -> Bus Creator/7  "ContactorPower"

== system BuckyWagon_01/Strategy/DataLogger Data ==
  Inputs : Inport  OutDataType=sfix(16)  OutScaling=2^0
  Outputs : Inport  Port=2  OutDataType=sfix(16)  OutScaling=2^0
  Bus Selector : BusSelector  OutputSignals=Virtual.VehicleSpeed,Physical.DC_Voltage,Virtual.BattOCV,Virtual.SOC
  Bus Selector1 : BusSelector  OutputSignals=Physical.Accel,Physical.BrakeSw,Physical.EStopSw,Physical.NLG5.pluggedIn,Physical.DC_Current
  Bus Selector3 : BusSelector  OutputSignals=Physical.BattTemp,Physical.LVVoltage
  Bus Selector4 : BusSelector  OutputSignals=InReverse
  Constant : Constant  Value=0  OutDataType=sfix(16)  OutScaling=2^0
  Constant1 : Constant  Value=0  OutDataType=sfix(16)  OutScaling=2^0
  Constant2 : Constant  Value=0  OutDataType=sfix(16)  OutScaling=2^0
  Embedded MATLAB Function : Stateflow chart  TreatAsAtomicUnit=on
  Send CAN Messages : MotoHawk_lib/CAN Blocks/Send CAN Messages  bus=-2  nam='CAN_2'  msgl=ARDAQ_200  pace=5  labelwires=off
  Send CAN Messages1 : MotoHawk_lib/CAN Blocks/Send CAN Messages  bus=-2  nam='CAN_2'  msgl=ARDAQ_201  pace=5  labelwires=off
  Send CAN Messages2 : MotoHawk_lib/CAN Blocks/Send CAN Messages  bus=-2  nam='CAN_2'  msgl=ARDAQ_202  pace=5  labelwires=off
  Send CAN Messages3 : MotoHawk_lib/CAN Blocks/Send CAN Messages  bus=-2  nam='CAN_2'  msgl=ARDAQ_203  pace=5  labelwires=off
  Send CAN Messages4 : MotoHawk_lib/CAN Blocks/Send CAN Messages  bus=-2  nam='CAN_2'  msgl=ARDAQ_204  pace=5  labelwires=off
  Send CAN Messages5 : MotoHawk_lib/CAN Blocks/Send CAN Messages  bus=-2  nam='CAN_2'  msgl=ARDAQ_205  pace=5  labelwires=off
  motohawk_data_read : MotoHawk_lib/Data Storage Blocks/motohawk_data_read  source=Lookup By Name  structure=Scalar  operation=Read scalar from location by index  sz_vec=4  sz_row=2  sz_col=3  typ=uint8  nam='cCOn'  checkNull=on  struct_inst_name=''  struct_nam='MyStruct'
  motohawk_data_read1 : MotoHawk_lib/Data Storage Blocks/motohawk_data_read  source=Lookup By Name  structure=Scalar  operation=Read scalar from location by index  sz_vec=4  sz_row=2  sz_col=3  typ=uint8  nam='ChargingState'  checkNull=on  struct_inst_name=''  struct_nam='MyStruct'
  motohawk_data_read2 : MotoHawk_lib/Data Storage Blocks/motohawk_data_read  source=Lookup By Name  structure=Scalar  operation=Read scalar from location by index  sz_vec=4  sz_row=2  sz_col=3  typ=double  nam='cCSpeedSet'  checkNull=on  struct_inst_name=''  struct_nam='MyStruct'
  motohawk_data_read3 : MotoHawk_lib/Data Storage Blocks/motohawk_data_read  source=Lookup By Name  structure=Scalar  operation=Read scalar from location by index  sz_vec=4  sz_row=2  sz_col=3  typ=uint32  nam='startupCount'  checkNull=on  struct_inst_name=''  struct_nam='MyStruct'
  motohawk_data_read4 : MotoHawk_lib/Data Storage Blocks/motohawk_data_read  source=Lookup By Name  structure=Scalar  operation=Read scalar from location by index  sz_vec=4  sz_row=2  sz_col=3  typ=uint32  nam='totalOnTime'  checkNull=on  struct_inst_name=''  struct_nam='MyStruct'
  motohawk_fault_statuses : MotoHawk_lib/Fault Management Blocks/motohawk_fault_statuses  nam=motohawk_get_faults(bdroot)  status=Active
  wires:
  Inputs/1 -> Bus Selector/1, Bus Selector1/1, Bus Selector3/1
  Bus Selector/1 -> Send CAN Messages1/1  "<VehicleSpeed>"
  Bus Selector/2 -> Send CAN Messages1/2  "<DC_Voltage>"
  motohawk_data_read/1 -> Send CAN Messages2/5
  Bus Selector1/1 -> Send CAN Messages2/1  "<Accel>"
  Bus Selector1/2 -> Send CAN Messages2/2  "<BrakeSw>"
  Bus Selector1/3 -> Send CAN Messages2/4  "<EStopSw>"
  Bus Selector1/4 -> Send CAN Messages2/6  "<pluggedIn>"
  Bus Selector1/5 -> Send CAN Messages2/8  "<DC_Current>"
  motohawk_data_read1/1 -> Send CAN Messages2/7
  Constant1/1 -> Send CAN Messages3/1, Send CAN Messages3/2, Send CAN Messages3/3, Send CAN Messages3/4, Send CAN Messages4/1
  Bus Selector3/1 -> Send CAN Messages4/2  "<BattTemp>"
  Bus Selector3/2 -> Send CAN Messages4/4  "<LVVoltage>"
  motohawk_data_read2/1 -> Send CAN Messages4/3
  motohawk_fault_statuses/1 -> Embedded MATLAB Function/1(faultStatus)
  Embedded MATLAB Function/1(fault1) -> Send CAN Messages5/1
  Embedded MATLAB Function/2(fault2) -> Send CAN Messages5/2
  motohawk_data_read3/1 -> Send CAN Messages/1
  motohawk_data_read4/1 -> Send CAN Messages/2
  Outputs/1 -> Bus Selector4/1
  Bus Selector4/1 -> Send CAN Messages2/3  "<InReverse>"
  Bus Selector/3 -> Send CAN Messages1/3  "<BattOCV>"
  Bus Selector/4 -> Send CAN Messages1/4  "<SOC>"
  Constant/1 -> Send CAN Messages2/10
  Constant2/1 -> Send CAN Messages2/9
